simulink model "ejercicio_1_4"  (R2017b)
settings: Solver=VariableStepAuto  StartTime=0.0  StopTime=0.2  RelTol=1e-3
libraries: dsparch4 x1
settings Model: Creator=Toti  LastModifiedBy=Toti
settings DataIOCC: LimitDataPoints=on  SaveOutput=off  SaveTime=off
settings OptimizationCC: BlockReduction=off  BooleanDataType=off  LifeSpan=inf
settings DebuggingCC: SaveWithParameterizedLinksMsg=none  UnderspecifiedInitializationDetection=Classic  MergeDetectMultiDrivingBlocksExec=none  SignalResolutionControl=TryResolveAllWithWarning  AllowSymbolicDim=off  SFUnexpectedBacktrackingDiag=warning  SFNoUnconditionalDefaultTransitionDiag=warning  SFExecutionAtInitializationDiag=none
settings HardwareCC: TargetUnknown=on
settings CodeAppCC: StateflowObjectComments=on
settings GRTTargetCC: TargetLangStandard=C89/C90 (ANSI)  GeneratePreprocessorConditionals=Disable all

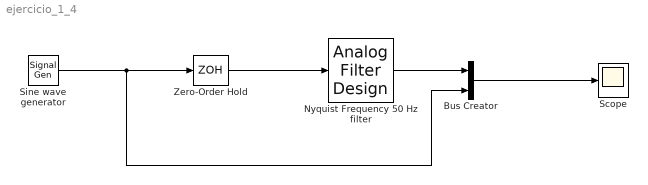
== system ejercicio_1_4 ==
  Bus Creator : BusCreator  Inputs=2
  Nyquist Frequency 50 Hz filter : dsparch4/Analog Filter Design  method=Butterworth  filttype=Lowpass  N=8  Wlo=314.16  Whi=80  Rp=2  Rs=40
  Scope : Scope
  Sine wave generator : SignalGenerator  Frequency=65
  "Zero-Order Hold " : ZeroOrderHold  SampleTime=0.01
  wires:
  "Zero-Order Hold "/1 -> Nyquist Frequency 50 Hz filter/1
  Nyquist Frequency 50 Hz filter/1 -> Bus Creator/1
  Bus Creator/1 -> Scope/1
  Sine wave generator/1 -> Bus Creator/2, "Zero-Order Hold "/1
